simulink model "ieee80211n"  (Simulink 6.0)
settings: Solver=VariableStepDiscrete  StartTime=0.0  StopTime=inf  RelTol=1e-3
PreLoadFcn:
  | load IEEE80211n_init;
values from neighbouring files (symbols this model uses):
  params =     [IEEE80211n_init.mat]    (also in IEEE80211n_settings.m = p)
undefined symbols (not defined in the file or in its folder): magnitude
libraries: commblkintrlv2 x196, dspsigops x143, simulink x136, commdigbbndam2 x98, dspmtrx3 x96, dspsigattribs x69, dspstat3 x38, commutil2 x32, commsequence2 x26, commcnvcod2 x10, dspindex x9, dspmlti3 x8
(part 5 of 12)

== system ieee80211n/ModulatorBank/ModulatorSS1 ==
  mode : Inport  Port=1  LatchInput=off
  txbits : Inport  Port=2  LatchInput=off
  Fcn2 : Fcn  Expr=u==1
  Fcn3 : Fcn  Expr=u==2
  Fcn4 : Fcn  Expr=u==3
  Fcn5 : Fcn  Expr=u==4
  Fcn6 : Fcn  Expr=u==5
  Fcn7 : Fcn  Expr=u==6
  Fcn8 : Fcn  Expr=u==7
  Fcn9 : Fcn  Expr=u==8
  Merge1 : Merge  Inputs=8
  Modulator 1 : Subsystem  AncestorBlock=IEEE80211a_lib/Modulator  TreatAsAtomicUnit=on  mask(QAM Modulator-Coder.){numSymbols=832, modulation=BPSK, code=1/2, trellisStructure=poly2trellis(7, [171 133]), punctureVector=[1]}
      mask prompts: numSymbols "Number of symbols per frame:"; trellisStructure "Trellis:"; punctureVector "Puncture vector:"
      mask help: Modulator gates incoming bits so that a bank of different modulators can share the same input frame size.
      mask init: same as ieee80211n/Demodbank/DecodeBankViterbi/Demodulator 2
      mask Display: disp(['Modulator\n' modulation ' ' code])
  Modulator 2 : Subsystem  AncestorBlock=IEEE80211a_lib/Modulator  TreatAsAtomicUnit=on  mask(QAM Modulator-Coder.){numSymbols=832, modulation=QPSK, code=1/2, trellisStructure=poly2trellis(7, [171 133]), punctureVector=[1]}
      mask prompts: numSymbols "Number of symbols per frame:"; trellisStructure "Trellis:"; punctureVector "Puncture vector:"
      mask help: Modulator gates incoming bits so that a bank of different modulators can share the same input frame size.
      mask init: same as ieee80211n/Demodbank/DecodeBankViterbi/Demodulator 2
      mask Display: disp(['Modulator\n' modulation ' ' code])
  Modulator 3 : Subsystem  AncestorBlock=IEEE80211a_lib/Modulator  TreatAsAtomicUnit=on  mask(QAM Modulator-Coder.){numSymbols=832, modulation=QPSK, code=3/4, trellisStructure=poly2trellis(7, [171 133]), punctureVector=[1 1 1 0 0 1].'}
      mask prompts: numSymbols "Number of symbols per frame:"; trellisStructure "Trellis:"; punctureVector "Puncture vector:"
      mask help: Modulator gates incoming bits so that a bank of different modulators can share the same input frame size.
      mask init: same as ieee80211n/Demodbank/DecodeBankViterbi/Demodulator 2
      mask Display: disp(['Modulator\n' modulation ' ' code])
  Modulator 4 : Subsystem  AncestorBlock=IEEE80211a_lib/Modulator  TreatAsAtomicUnit=on  mask(QAM Modulator-Coder.){numSymbols=832, modulation=16-QAM, code=1/2, trellisStructure=poly2trellis(7, [171 133]), punctureVector=[1]}
      mask prompts: numSymbols "Number of symbols per frame:"; trellisStructure "Trellis:"; punctureVector "Puncture vector:"
      mask help: Modulator gates incoming bits so that a bank of different modulators can share the same input frame size.
      mask init: same as ieee80211n/Demodbank/DecodeBankViterbi/Demodulator 2
      mask Display: disp(['Modulator\n' modulation ' ' code])
  Modulator 5 : Subsystem  AncestorBlock=IEEE80211a_lib/Modulator  TreatAsAtomicUnit=on  mask(QAM Modulator-Coder.){numSymbols=832, modulation=16-QAM, code=3/4, trellisStructure=poly2trellis(7, [171 133]), punctureVector=[1 1 1 0 0 1].'}
      mask prompts: numSymbols "Number of symbols per frame:"; trellisStructure "Trellis:"; punctureVector "Puncture vector:"
      mask help: Modulator gates incoming bits so that a bank of different modulators can share the same input frame size.
      mask init:
      | % number of bits per symbol
      | switch modulation
      | 	case 'BPSK', Nb1 = 1;
      | 	case 'QPSK', Nb1 = 2;
      | 	case '16-QAM', Nb1 = 4;
      | 	case '64-QAM', Nb1 = 6;
      | end
      | 
      | modOrder = 2.^Nb1;
      | Nb = numSymbols * Nb1; % tx bits per block
      | codeRate = str2num(strvcat(code)).';
      | bitsPerBlock = Nb .* codeRate;
      | 
      | % interleaver
      | interleaverRows = 13;
      | if rem(Nb, interleaverRows)
      | 	error('Number of transmitted bits per block must be multiple of 16.')
      | end
      | interleaverCols = Nb / interleaverRows;
      | interleaverElements = [...
      |             2*floor( [0:Nb-1]/2 ) + ...
      |             mod( ([0:Nb-1] + Nb - floor( interleaverRows*[0:Nb-1]/Nb ) ), 2 ) ...
      |             + 1]';
      mask Display: disp(['Modulator\n' modulation ' ' code])
  Modulator 6 : Subsystem  AncestorBlock=IEEE80211a_lib/Modulator  TreatAsAtomicUnit=on  mask(QAM Modulator-Coder.){numSymbols=832, modulation=64-QAM, code=2/3, trellisStructure=poly2trellis(7, [133 171]), punctureVector=[1 1 1 0].'}
      mask prompts: numSymbols "Number of symbols per frame:"; trellisStructure "Trellis:"; punctureVector "Puncture vector:"
      mask help: Modulator gates incoming bits so that a bank of different modulators can share the same input frame size.
      mask init: same as ieee80211n/Demodbank/DecodeBankViterbi/Demodulator 2
      mask Display: disp(['Modulator\n' modulation ' ' code])
  Modulator 7 : Subsystem  AncestorBlock=IEEE80211a_lib/Modulator  TreatAsAtomicUnit=on  mask(QAM Modulator-Coder.){numSymbols=832, modulation=64-QAM, code=3/4, trellisStructure=poly2trellis(7, [133 171]), punctureVector=[1 1 1 0 0 1].'}
      mask prompts: numSymbols "Number of symbols per frame:"; trellisStructure "Trellis:"; punctureVector "Puncture vector:"
      mask help: Modulator gates incoming bits so that a bank of different modulators can share the same input frame size.
      mask init: same as ieee80211n/Demodbank/DecodeBankViterbi/Demodulator 1
      mask Display: disp(['Modulator\n' modulation ' ' code])
  Modulator 8 : Subsystem  AncestorBlock=IEEE80211a_lib/Modulator  TreatAsAtomicUnit=on  mask(QAM Modulator-Coder.){numSymbols=832, modulation=64-QAM, code=5/6, trellisStructure=poly2trellis(7, [133 171]), punctureVector=[1 1 1 0 0 1 1 0 0 1].'}
      mask prompts: numSymbols "Number of symbols per frame:"; trellisStructure "Trellis:"; punctureVector "Puncture vector:"
      mask help: Modulator gates incoming bits so that a bank of different modulators can share the same input frame size.
      mask init: same as ieee80211n/Demodbank/DecodeBankViterbi/Demodulator 2
      mask Display: disp(['Modulator\n' modulation ' ' code])
  sig : Outport
  wires:
  Merge1/1 -> sig/1
  mode/1 -> Fcn2/1, Fcn7/1, Fcn8/1, Fcn9/1, Fcn6/1, Fcn5/1, Fcn4/1, Fcn3/1
  txbits/1 -> Modulator 1/1(txdata), Modulator 6/1(txdata), Modulator 7/1(txdata), Modulator 8/1(txdata), Modulator 5/1(txdata), Modulator 4/1(txdata), Modulator 3/1(txdata), Modulator 2/1(txdata)
  Modulator 1/1(txsig) -> Merge1/1
  Modulator 2/1(txsig) -> Merge1/2
  Modulator 3/1(txsig) -> Merge1/3
  Modulator 4/1(txsig) -> Merge1/4
  Modulator 5/1(txsig) -> Merge1/5
  Modulator 6/1(txsig) -> Merge1/6
  Modulator 7/1(txsig) -> Merge1/7
  Fcn2/1 -> Modulator 1/Enable
  Fcn3/1 -> Modulator 2/Enable
  Fcn4/1 -> Modulator 3/Enable
  Fcn5/1 -> Modulator 4/Enable
  Fcn6/1 -> Modulator 5/Enable
  Fcn7/1 -> Modulator 6/Enable
  Fcn8/1 -> Modulator 7/Enable
  Fcn9/1 -> Modulator 8/Enable
  Modulator 8/1(txsig) -> Merge1/8

== system ieee80211n/ModulatorBank/ModulatorSS2 ==
  mode : Inport  Port=1  LatchInput=off
  txbits : Inport  Port=2  LatchInput=off
  Fcn2 : Fcn  Expr=u==1
  Fcn3 : Fcn  Expr=u==2
  Fcn4 : Fcn  Expr=u==3
  Fcn5 : Fcn  Expr=u==4
  Fcn6 : Fcn  Expr=u==5
  Fcn7 : Fcn  Expr=u==6
  Fcn8 : Fcn  Expr=u==7
  Fcn9 : Fcn  Expr=u==8
  Merge1 : Merge  Inputs=8
  Modulator 1 : Subsystem  AncestorBlock=IEEE80211a_lib/Modulator  TreatAsAtomicUnit=on  mask(QAM Modulator-Coder.){numSymbols=832, modulation=BPSK, code=1/2, trellisStructure=poly2trellis(7, [171 133]), punctureVector=[1]}
      mask prompts: numSymbols "Number of symbols per frame:"; trellisStructure "Trellis:"; punctureVector "Puncture vector:"
      mask help: Modulator gates incoming bits so that a bank of different modulators can share the same input frame size.
      mask init:
      | % number of bits per symbol
      | switch modulation
      | 	case 'BPSK', Nb1 = 1;
      | 	case 'QPSK', Nb1 = 2;
      | 	case '16-QAM', Nb1 = 4;
      | 	case '64-QAM', Nb1 = 6;
      | end
      | 
      | modOrder = 2.^Nb1;
      | Nb = numSymbols * Nb1; % tx bits per block
      | codeRate = str2num(strvcat(code)).';
      | bitsPerBlock = Nb .* codeRate;
      | s=max([Nb1/2 1]);
      | 
      | % interleaver
      | interleaverRows = 13;
      | if rem(Nb, interleaverRows)
      | 	error('Number of transmitted bits per block must be multiple of 16.')
      | end
      | interleaverCols = Nb / interleaverRows;
      | interleaverElements = [...
      |             s*floor( [0:Nb-1]/s ) + ...
      |             mod( ([0:Nb-1] + Nb - floor( interleaverRows*[0:Nb-1]/Nb ) ), s ) ...
      |             + 1]';
      | 	
      | if 1 %%%%%%%%%%%%%%%%%%%%%%%%
      | % freq rotation interleaver
      | iss = 1;
      | freqRotNum = 2*11;  % 20MHz channel
      | freqRotInterleaverElements = [...
      |             mod([0:Nb-1] - (mod(2*iss, 3) + 3*floor(iss/3)*freqRotNum*Nb1), Nb) ...
      |             + 1]';
      | end   %%%%%%%%%%%%%%%%%%%%%%%%
      mask Display: disp(['Modulator\n' modulation ' ' code])
  Modulator 2 : Subsystem  AncestorBlock=IEEE80211a_lib/Modulator  TreatAsAtomicUnit=on  mask(QAM Modulator-Coder.){numSymbols=832, modulation=QPSK, code=1/2, trellisStructure=poly2trellis(7, [171 133]), punctureVector=[1]}
      mask prompts: numSymbols "Number of symbols per frame:"; trellisStructure "Trellis:"; punctureVector "Puncture vector:"
      mask help: Modulator gates incoming bits so that a bank of different modulators can share the same input frame size.
      mask init: same as ieee80211n/Demodbank/Demod_ss2/Demodulator 1
      mask Display: disp(['Modulator\n' modulation ' ' code])
  Modulator 3 : Subsystem  AncestorBlock=IEEE80211a_lib/Modulator  TreatAsAtomicUnit=on  mask(QAM Modulator-Coder.){numSymbols=832, modulation=QPSK, code=3/4, trellisStructure=poly2trellis(7, [171 133]), punctureVector=[1 1 1 0 0 1].'}
      mask prompts: numSymbols "Number of symbols per frame:"; trellisStructure "Trellis:"; punctureVector "Puncture vector:"
      mask help: Modulator gates incoming bits so that a bank of different modulators can share the same input frame size.
      mask init: same as ieee80211n/Demodbank/Demod_ss2/Demodulator 1
      mask Display: disp(['Modulator\n' modulation ' ' code])
  Modulator 4 : Subsystem  AncestorBlock=IEEE80211a_lib/Modulator  TreatAsAtomicUnit=on  mask(QAM Modulator-Coder.){numSymbols=832, modulation=16-QAM, code=1/2, trellisStructure=poly2trellis(7, [171 133]), punctureVector=[1]}
      mask prompts: numSymbols "Number of symbols per frame:"; trellisStructure "Trellis:"; punctureVector "Puncture vector:"
      mask help: Modulator gates incoming bits so that a bank of different modulators can share the same input frame size.
      mask init: same as ieee80211n/Demodbank/Demod_ss2/Demodulator 1
      mask Display: disp(['Modulator\n' modulation ' ' code])
  Modulator 5 : Subsystem  AncestorBlock=IEEE80211a_lib/Modulator  TreatAsAtomicUnit=on  mask(QAM Modulator-Coder.){numSymbols=832, modulation=16-QAM, code=3/4, trellisStructure=poly2trellis(7, [171 133]), punctureVector=[1 1 1 0 0 1].'}
      mask prompts: numSymbols "Number of symbols per frame:"; trellisStructure "Trellis:"; punctureVector "Puncture vector:"
      mask help: Modulator gates incoming bits so that a bank of different modulators can share the same input frame size.
      mask init: same as ieee80211n/Demodbank/Demod_ss2/Demodulator 1
      mask Display: disp(['Modulator\n' modulation ' ' code])
  Modulator 6 : Subsystem  AncestorBlock=IEEE80211a_lib/Modulator  TreatAsAtomicUnit=on  mask(QAM Modulator-Coder.){numSymbols=832, modulation=64-QAM, code=2/3, trellisStructure=poly2trellis(7, [133 171]), punctureVector=[1 1 1 0].'}
      mask prompts: numSymbols "Number of symbols per frame:"; trellisStructure "Trellis:"; punctureVector "Puncture vector:"
      mask help: Modulator gates incoming bits so that a bank of different modulators can share the same input frame size.
      mask init: same as ieee80211n/Demodbank/Demod_ss2/Demodulator 1
      mask Display: disp(['Modulator\n' modulation ' ' code])
  Modulator 7 : Subsystem  AncestorBlock=IEEE80211a_lib/Modulator  TreatAsAtomicUnit=on  mask(QAM Modulator-Coder.){numSymbols=832, modulation=64-QAM, code=3/4, trellisStructure=poly2trellis(7, [133 171]), punctureVector=[1 1 1 0 0 1].'}
      mask prompts: numSymbols "Number of symbols per frame:"; trellisStructure "Trellis:"; punctureVector "Puncture vector:"
      mask help: Modulator gates incoming bits so that a bank of different modulators can share the same input frame size.
      mask init: same as ieee80211n/Demodbank/Demod_ss2/Demodulator 1
      mask Display: disp(['Modulator\n' modulation ' ' code])
  Modulator 8 : Subsystem  AncestorBlock=IEEE80211a_lib/Modulator  TreatAsAtomicUnit=on  mask(QAM Modulator-Coder.){numSymbols=832, modulation=64-QAM, code=5/6, trellisStructure=poly2trellis(7, [133 171]), punctureVector=[1 1 1 0 0 1 1 0 0 1].'}
      mask prompts: numSymbols "Number of symbols per frame:"; trellisStructure "Trellis:"; punctureVector "Puncture vector:"
      mask help: Modulator gates incoming bits so that a bank of different modulators can share the same input frame size.
      mask init:
      | % number of bits per symbol
      | switch modulation
      | 	case 'BPSK', Nb1 = 1;
      | 	case 'QPSK', Nb1 = 2;
      | 	case '16-QAM', Nb1 = 4;
      | 	case '64-QAM', Nb1 = 6;
      | 	case '256-QAM', Nb1 = 8;
      | end
      | 
      | modOrder = 2.^Nb1;
      | Nb = numSymbols * Nb1; % tx bits per block
      | codeRate = str2num(strvcat(code)).';
      | bitsPerBlock = Nb .* codeRate;
      | s=max([Nb1/2 1]);
      | 
      | % interleaver
      | interleaverRows = 13;
      | if rem(Nb, interleaverRows)
      | 	error('Number of transmitted bits per block must be multiple of 16.')
      | end
      | interleaverCols = Nb / interleaverRows;
      | interleaverElements = [...
      |             s*floor( [0:Nb-1]/s ) + ...
      |             mod( ([0:Nb-1] + Nb - floor( interleaverRows*[0:Nb-1]/Nb ) ), s ) ...
      |             + 1]';
      | 	
      | if 1 %%%%%%%%%%%%%%%%%%%%%%%%
      | % freq rotation interleaver
      | iss = 1;
      | freqRotNum = 2*11;  % 20MHz channel
      | freqRotInterleaverElements = [...
      |             mod([0:Nb-1] - (mod(2*iss, 3) + 3*floor(iss/3)*freqRotNum*Nb1), Nb) ...
      |             + 1]';
      | end   %%%%%%%%%%%%%%%%%%%%%%%%
      mask Display: disp(['Modulator\n' modulation ' ' code])
  sig : Outport
  wires:
  Merge1/1 -> sig/1
  mode/1 -> Fcn2/1, Fcn7/1, Fcn8/1, Fcn9/1, Fcn6/1, Fcn5/1, Fcn4/1, Fcn3/1
  txbits/1 -> Modulator 1/1(txdata), Modulator 6/1(txdata), Modulator 7/1(txdata), Modulator 8/1(txdata), Modulator 5/1(txdata), Modulator 4/1(txdata), Modulator 3/1(txdata), Modulator 2/1(txdata)
  Modulator 1/1(txsig) -> Merge1/1
  Modulator 2/1(txsig) -> Merge1/2
  Modulator 3/1(txsig) -> Merge1/3
  Modulator 4/1(txsig) -> Merge1/4
  Modulator 5/1(txsig) -> Merge1/5
  Modulator 6/1(txsig) -> Merge1/6
  Modulator 7/1(txsig) -> Merge1/7
  Fcn2/1 -> Modulator 1/Enable
  Fcn3/1 -> Modulator 2/Enable
  Fcn4/1 -> Modulator 3/Enable
  Fcn5/1 -> Modulator 4/Enable
  Fcn6/1 -> Modulator 5/Enable
  Fcn7/1 -> Modulator 6/Enable
  Fcn8/1 -> Modulator 7/Enable
  Fcn9/1 -> Modulator 8/Enable
  Modulator 8/1(txsig) -> Merge1/8

== system ieee80211n/ModulatorBank/ModulatorSS3 ==
  mode : Inport  Port=1  LatchInput=off
  txbits : Inport  Port=2  LatchInput=off
  Fcn2 : Fcn  Expr=u==1
  Fcn3 : Fcn  Expr=u==2
  Fcn4 : Fcn  Expr=u==3
  Fcn5 : Fcn  Expr=u==4
  Fcn6 : Fcn  Expr=u==5
  Fcn7 : Fcn  Expr=u==6
  Fcn8 : Fcn  Expr=u==7
  Fcn9 : Fcn  Expr=u==8
  Merge1 : Merge  Inputs=8
  Modulator 1 : Subsystem  AncestorBlock=IEEE80211a_lib/Modulator  TreatAsAtomicUnit=on  mask(QAM Modulator-Coder.){numSymbols=832, modulation=BPSK, code=1/2, trellisStructure=poly2trellis(7, [171 133]), punctureVector=[1]}
      mask prompts: numSymbols "Number of symbols per frame:"; trellisStructure "Trellis:"; punctureVector "Puncture vector:"
      mask help: Modulator gates incoming bits so that a bank of different modulators can share the same input frame size.
      mask init:
      | % number of bits per symbol
      | switch modulation
      | 	case 'BPSK', Nb1 = 1;
      | 	case 'QPSK', Nb1 = 2;
      | 	case '16-QAM', Nb1 = 4;
      | 	case '64-QAM', Nb1 = 6;
      | end
      | 
      | modOrder = 2.^Nb1;
      | Nb = numSymbols * Nb1; % tx bits per block
      | codeRate = str2num(strvcat(code)).';
      | bitsPerBlock = Nb .* codeRate;
      | s=max([Nb1/2 1]);
      | 
      | % interleaver
      | interleaverRows = 13;
      | if rem(Nb, interleaverRows)
      | 	error('Number of transmitted bits per block must be multiple of 16.')
      | end
      | interleaverCols = Nb / interleaverRows;
      | interleaverElements = [...
      |             s*floor( [0:Nb-1]/s ) + ...
      |             mod( ([0:Nb-1] + Nb - floor( interleaverRows*[0:Nb-1]/Nb ) ), s ) ...
      |             + 1]';
      | 	
      | if 1 %%%%%%%%%%%%%%%%%%%%%%%%
      | % freq rotation interleaver
      | iss = 2;
      | freqRotNum = 1*11;  % 20MHz channel
      | freqRotInterleaverElements = [...
      |             mod([0:Nb-1] - (mod(2*iss, 3) + 3*floor(iss/3)*freqRotNum*Nb1), Nb) ...
      |             + 1]';
      | end   %%%%%%%%%%%%%%%%%%%%%%%%
      mask Display: disp(['Modulator\n' modulation ' ' code])
  Modulator 2 : Subsystem  AncestorBlock=IEEE80211a_lib/Modulator  TreatAsAtomicUnit=on  mask(QAM Modulator-Coder.){numSymbols=832, modulation=QPSK, code=1/2, trellisStructure=poly2trellis(7, [171 133]), punctureVector=[1]}
      mask prompts: numSymbols "Number of symbols per frame:"; trellisStructure "Trellis:"; punctureVector "Puncture vector:"
      mask help: Modulator gates incoming bits so that a bank of different modulators can share the same input frame size.
      mask init: same as ieee80211n/ModulatorBank/ModulatorSS3/Modulator 1
      mask Display: disp(['Modulator\n' modulation ' ' code])
  Modulator 3 : Subsystem  AncestorBlock=IEEE80211a_lib/Modulator  TreatAsAtomicUnit=on  mask(QAM Modulator-Coder.){numSymbols=832, modulation=QPSK, code=3/4, trellisStructure=poly2trellis(7, [171 133]), punctureVector=[1 1 1 0 0 1].'}
      mask prompts: numSymbols "Number of symbols per frame:"; trellisStructure "Trellis:"; punctureVector "Puncture vector:"
      mask help: Modulator gates incoming bits so that a bank of different modulators can share the same input frame size.
      mask init: same as ieee80211n/ModulatorBank/ModulatorSS3/Modulator 1
      mask Display: disp(['Modulator\n' modulation ' ' code])
  Modulator 4 : Subsystem  AncestorBlock=IEEE80211a_lib/Modulator  TreatAsAtomicUnit=on  mask(QAM Modulator-Coder.){numSymbols=832, modulation=16-QAM, code=1/2, trellisStructure=poly2trellis(7, [171 133]), punctureVector=[1]}
      mask prompts: numSymbols "Number of symbols per frame:"; trellisStructure "Trellis:"; punctureVector "Puncture vector:"
      mask help: Modulator gates incoming bits so that a bank of different modulators can share the same input frame size.
      mask init: same as ieee80211n/ModulatorBank/ModulatorSS3/Modulator 1
      mask Display: disp(['Modulator\n' modulation ' ' code])
  Modulator 5 : Subsystem  AncestorBlock=IEEE80211a_lib/Modulator  TreatAsAtomicUnit=on  mask(QAM Modulator-Coder.){numSymbols=832, modulation=16-QAM, code=3/4, trellisStructure=poly2trellis(7, [171 133]), punctureVector=[1 1 1 0 0 1].'}
      mask prompts: numSymbols "Number of symbols per frame:"; trellisStructure "Trellis:"; punctureVector "Puncture vector:"
      mask help: Modulator gates incoming bits so that a bank of different modulators can share the same input frame size.
      mask init: same as ieee80211n/ModulatorBank/ModulatorSS3/Modulator 1
      mask Display: disp(['Modulator\n' modulation ' ' code])
  Modulator 6 : Subsystem  AncestorBlock=IEEE80211a_lib/Modulator  TreatAsAtomicUnit=on  mask(QAM Modulator-Coder.){numSymbols=832, modulation=64-QAM, code=2/3, trellisStructure=poly2trellis(7, [133 171]), punctureVector=[1 1 1 0].'}
      mask prompts: numSymbols "Number of symbols per frame:"; trellisStructure "Trellis:"; punctureVector "Puncture vector:"
      mask help: Modulator gates incoming bits so that a bank of different modulators can share the same input frame size.
      mask init: same as ieee80211n/ModulatorBank/ModulatorSS3/Modulator 1
      mask Display: disp(['Modulator\n' modulation ' ' code])
  Modulator 7 : Subsystem  AncestorBlock=IEEE80211a_lib/Modulator  TreatAsAtomicUnit=on  mask(QAM Modulator-Coder.){numSymbols=832, modulation=64-QAM, code=3/4, trellisStructure=poly2trellis(7, [133 171]), punctureVector=[1 1 1 0 0 1].'}
      mask prompts: numSymbols "Number of symbols per frame:"; trellisStructure "Trellis:"; punctureVector "Puncture vector:"
      mask help: Modulator gates incoming bits so that a bank of different modulators can share the same input frame size.
      mask init: same as ieee80211n/ModulatorBank/ModulatorSS3/Modulator 1
      mask Display: disp(['Modulator\n' modulation ' ' code])
  Modulator 8 : Subsystem  AncestorBlock=IEEE80211a_lib/Modulator  TreatAsAtomicUnit=on  mask(QAM Modulator-Coder.){numSymbols=832, modulation=64-QAM, code=5/6, trellisStructure=poly2trellis(7, [133 171]), punctureVector=[1 1 1 0 0 1 1 0 0 1].'}
      mask prompts: numSymbols "Number of symbols per frame:"; trellisStructure "Trellis:"; punctureVector "Puncture vector:"
      mask help: Modulator gates incoming bits so that a bank of different modulators can share the same input frame size.
      mask init:
      | % number of bits per symbol
      | switch modulation
      | 	case 'BPSK', Nb1 = 1;
      | 	case 'QPSK', Nb1 = 2;
      | 	case '16-QAM', Nb1 = 4;
      | 	case '64-QAM', Nb1 = 6;
      | 	case '256-QAM', Nb1 = 8;
      | end
      | 
      | modOrder = 2.^Nb1;
      | Nb = numSymbols * Nb1; % tx bits per block
      | codeRate = str2num(strvcat(code)).';
      | bitsPerBlock = Nb .* codeRate;
      | s=max([Nb1/2 1]);
      | 
      | % interleaver
      | interleaverRows = 13;
      | if rem(Nb, interleaverRows)
      | 	error('Number of transmitted bits per block must be multiple of 16.')
      | end
      | interleaverCols = Nb / interleaverRows;
      | interleaverElements = [...
      |             s*floor( [0:Nb-1]/s ) + ...
      |             mod( ([0:Nb-1] + Nb - floor( interleaverRows*[0:Nb-1]/Nb ) ), s ) ...
      |             + 1]';
      | 	
      | if 1 %%%%%%%%%%%%%%%%%%%%%%%%
      | % freq rotation interleaver
      | iss = 2;
      | freqRotNum = 1*11;  % 20MHz channel
      | freqRotInterleaverElements = [...
      |             mod([0:Nb-1] - (mod(2*iss, 3) + 3*floor(iss/3)*freqRotNum*Nb1), Nb) ...
      |             + 1]';
      | end   %%%%%%%%%%%%%%%%%%%%%%%%
      mask Display: disp(['Modulator\n' modulation ' ' code])
  sig : Outport
  wires:
  Merge1/1 -> sig/1
  mode/1 -> Fcn2/1, Fcn7/1, Fcn8/1, Fcn9/1, Fcn6/1, Fcn5/1, Fcn4/1, Fcn3/1
  txbits/1 -> Modulator 1/1(txdata), Modulator 6/1(txdata), Modulator 7/1(txdata), Modulator 8/1(txdata), Modulator 5/1(txdata), Modulator 4/1(txdata), Modulator 3/1(txdata), Modulator 2/1(txdata)
  Modulator 1/1(txsig) -> Merge1/1
  Modulator 2/1(txsig) -> Merge1/2
  Modulator 3/1(txsig) -> Merge1/3
  Modulator 4/1(txsig) -> Merge1/4
  Modulator 5/1(txsig) -> Merge1/5
  Modulator 6/1(txsig) -> Merge1/6
  Modulator 7/1(txsig) -> Merge1/7
  Fcn2/1 -> Modulator 1/Enable
  Fcn3/1 -> Modulator 2/Enable
  Fcn4/1 -> Modulator 3/Enable
  Fcn5/1 -> Modulator 4/Enable
  Fcn6/1 -> Modulator 5/Enable
  Fcn7/1 -> Modulator 6/Enable
  Fcn8/1 -> Modulator 7/Enable
  Fcn9/1 -> Modulator 8/Enable
  Modulator 8/1(txsig) -> Merge1/8

== system ieee80211n/ModulatorBank/ModulatorSS4 ==
  mode : Inport  Port=1  LatchInput=off
  txbits : Inport  Port=2  LatchInput=off
  Fcn2 : Fcn  Expr=u==1
  Fcn3 : Fcn  Expr=u==2
  Fcn4 : Fcn  Expr=u==3
  Fcn5 : Fcn  Expr=u==4
  Fcn6 : Fcn  Expr=u==5
  Fcn7 : Fcn  Expr=u==6
  Fcn8 : Fcn  Expr=u==7
  Fcn9 : Fcn  Expr=u==8
  Merge1 : Merge  Inputs=8
  Modulator 1 : Subsystem  AncestorBlock=IEEE80211a_lib/Modulator  TreatAsAtomicUnit=on  mask(QAM Modulator-Coder.){numSymbols=832, modulation=BPSK, code=1/2, trellisStructure=poly2trellis(7, [171 133]), punctureVector=[1]}
      mask prompts: numSymbols "Number of symbols per frame:"; trellisStructure "Trellis:"; punctureVector "Puncture vector:"
      mask help: Modulator gates incoming bits so that a bank of different modulators can share the same input frame size.
      mask init:
      | % number of bits per symbol
      | switch modulation
      | 	case 'BPSK', Nb1 = 1;
      | 	case 'QPSK', Nb1 = 2;
      | 	case '16-QAM', Nb1 = 4;
      | 	case '64-QAM', Nb1 = 6;
      | end
      | 
      | modOrder = 2.^Nb1;
      | Nb = numSymbols * Nb1; % tx bits per block
      | codeRate = str2num(strvcat(code)).';
      | bitsPerBlock = Nb .* codeRate;
      | s=max([Nb1/2 1]);
      | 
      | % interleaver
      | interleaverRows = 13;
      | if rem(Nb, interleaverRows)
      | 	error('Number of transmitted bits per block must be multiple of 16.')
      | end
      | interleaverCols = Nb / interleaverRows;
      | interleaverElements = [...
      |             s*floor( [0:Nb-1]/s ) + ...
      |             mod( ([0:Nb-1] + Nb - floor( interleaverRows*[0:Nb-1]/Nb ) ), s ) ...
      |             + 1]';
      | 	
      | if 1 %%%%%%%%%%%%%%%%%%%%%%%%
      | % freq rotation interleaver
      | iss = 3;
      | freqRotNum = 3*11;  % 20MHz channel
      | freqRotInterleaverElements = [...
      |             mod([0:Nb-1] - (mod(2*iss, 3) + 3*floor(iss/3)*freqRotNum*Nb1), Nb) ...
      |             + 1]';
      | end   %%%%%%%%%%%%%%%%%%%%%%%%
      mask Display: disp(['Modulator\n' modulation ' ' code])
  Modulator 2 : Subsystem  AncestorBlock=IEEE80211a_lib/Modulator  TreatAsAtomicUnit=on  mask(QAM Modulator-Coder.){numSymbols=832, modulation=QPSK, code=1/2, trellisStructure=poly2trellis(7, [171 133]), punctureVector=[1]}
      mask prompts: numSymbols "Number of symbols per frame:"; trellisStructure "Trellis:"; punctureVector "Puncture vector:"
      mask help: Modulator gates incoming bits so that a bank of different modulators can share the same input frame size.
      mask init: same as ieee80211n/Demodbank/Demod_ss4/Demodulator 1
      mask Display: disp(['Modulator\n' modulation ' ' code])
  Modulator 3 : Subsystem  AncestorBlock=IEEE80211a_lib/Modulator  TreatAsAtomicUnit=on  mask(QAM Modulator-Coder.){numSymbols=832, modulation=QPSK, code=3/4, trellisStructure=poly2trellis(7, [171 133]), punctureVector=[1 1 1 0 0 1].'}
      mask prompts: numSymbols "Number of symbols per frame:"; trellisStructure "Trellis:"; punctureVector "Puncture vector:"
      mask help: Modulator gates incoming bits so that a bank of different modulators can share the same input frame size.
      mask init: same as ieee80211n/Demodbank/Demod_ss4/Demodulator 1
      mask Display: disp(['Modulator\n' modulation ' ' code])
  Modulator 4 : Subsystem  AncestorBlock=IEEE80211a_lib/Modulator  TreatAsAtomicUnit=on  mask(QAM Modulator-Coder.){numSymbols=832, modulation=16-QAM, code=1/2, trellisStructure=poly2trellis(7, [171 133]), punctureVector=[1]}
      mask prompts: numSymbols "Number of symbols per frame:"; trellisStructure "Trellis:"; punctureVector "Puncture vector:"
      mask help: Modulator gates incoming bits so that a bank of different modulators can share the same input frame size.
      mask init: same as ieee80211n/Demodbank/Demod_ss4/Demodulator 1
      mask Display: disp(['Modulator\n' modulation ' ' code])
  Modulator 5 : Subsystem  AncestorBlock=IEEE80211a_lib/Modulator  TreatAsAtomicUnit=on  mask(QAM Modulator-Coder.){numSymbols=832, modulation=16-QAM, code=3/4, trellisStructure=poly2trellis(7, [171 133]), punctureVector=[1 1 1 0 0 1].'}
      mask prompts: numSymbols "Number of symbols per frame:"; trellisStructure "Trellis:"; punctureVector "Puncture vector:"
      mask help: Modulator gates incoming bits so that a bank of different modulators can share the same input frame size.
      mask init: same as ieee80211n/Demodbank/Demod_ss4/Demodulator 1
      mask Display: disp(['Modulator\n' modulation ' ' code])
  Modulator 6 : Subsystem  AncestorBlock=IEEE80211a_lib/Modulator  TreatAsAtomicUnit=on  mask(QAM Modulator-Coder.){numSymbols=832, modulation=64-QAM, code=2/3, trellisStructure=poly2trellis(7, [133 171]), punctureVector=[1 1 1 0].'}
      mask prompts: numSymbols "Number of symbols per frame:"; trellisStructure "Trellis:"; punctureVector "Puncture vector:"
      mask help: Modulator gates incoming bits so that a bank of different modulators can share the same input frame size.
      mask init: same as ieee80211n/Demodbank/Demod_ss4/Demodulator 1
      mask Display: disp(['Modulator\n' modulation ' ' code])
  Modulator 7 : Subsystem  AncestorBlock=IEEE80211a_lib/Modulator  TreatAsAtomicUnit=on  mask(QAM Modulator-Coder.){numSymbols=832, modulation=64-QAM, code=3/4, trellisStructure=poly2trellis(7, [133 171]), punctureVector=[1 1 1 0 0 1].'}
      mask prompts: numSymbols "Number of symbols per frame:"; trellisStructure "Trellis:"; punctureVector "Puncture vector:"
      mask help: Modulator gates incoming bits so that a bank of different modulators can share the same input frame size.
      mask init: same as ieee80211n/Demodbank/Demod_ss4/Demodulator 1
      mask Display: disp(['Modulator\n' modulation ' ' code])
  Modulator 8 : Subsystem  AncestorBlock=IEEE80211a_lib/Modulator  TreatAsAtomicUnit=on  mask(QAM Modulator-Coder.){numSymbols=832, modulation=64-QAM, code=5/6, trellisStructure=poly2trellis(7, [133 171]), punctureVector=[1 1 1 0 0 1 1 0 0 1].'}
      mask prompts: numSymbols "Number of symbols per frame:"; trellisStructure "Trellis:"; punctureVector "Puncture vector:"
      mask help: Modulator gates incoming bits so that a bank of different modulators can share the same input frame size.
      mask init:
      | % number of bits per symbol
      | switch modulation
      | 	case 'BPSK', Nb1 = 1;
      | 	case 'QPSK', Nb1 = 2;
      | 	case '16-QAM', Nb1 = 4;
      | 	case '64-QAM', Nb1 = 6;
      | 	case '256-QAM', Nb1 = 8;
      | end
      | 
      | modOrder = 2.^Nb1;
      | Nb = numSymbols * Nb1; % tx bits per block
      | codeRate = str2num(strvcat(code)).';
      | bitsPerBlock = Nb .* codeRate;
      | s=max([Nb1/2 1]);
      | 
      | % interleaver
      | interleaverRows = 13;
      | if rem(Nb, interleaverRows)
      | 	error('Number of transmitted bits per block must be multiple of 16.')
      | end
      | interleaverCols = Nb / interleaverRows;
      | interleaverElements = [...
      |             s*floor( [0:Nb-1]/s ) + ...
      |             mod( ([0:Nb-1] + Nb - floor( interleaverRows*[0:Nb-1]/Nb ) ), s ) ...
      |             + 1]';
      | 	
      | if 1 %%%%%%%%%%%%%%%%%%%%%%%%
      | % freq rotation interleaver
      | iss = 3;
      | freqRotNum = 3*11;  % 20MHz channel
      | freqRotInterleaverElements = [...
      |             mod([0:Nb-1] - (mod(2*iss, 3) + 3*floor(iss/3)*freqRotNum*Nb1), Nb) ...
      |             + 1]';
      | end   %%%%%%%%%%%%%%%%%%%%%%%%
      mask Display: disp(['Modulator\n' modulation ' ' code])
  sig : Outport
  wires:
  Merge1/1 -> sig/1
  mode/1 -> Fcn2/1, Fcn7/1, Fcn8/1, Fcn9/1, Fcn6/1, Fcn5/1, Fcn4/1, Fcn3/1
  txbits/1 -> Modulator 1/1(txdata), Modulator 6/1(txdata), Modulator 7/1(txdata), Modulator 8/1(txdata), Modulator 5/1(txdata), Modulator 4/1(txdata), Modulator 3/1(txdata), Modulator 2/1(txdata)
  Modulator 1/1(txsig) -> Merge1/1
  Modulator 2/1(txsig) -> Merge1/2
  Modulator 3/1(txsig) -> Merge1/3
  Modulator 4/1(txsig) -> Merge1/4
  Modulator 5/1(txsig) -> Merge1/5
  Modulator 6/1(txsig) -> Merge1/6
  Modulator 7/1(txsig) -> Merge1/7
  Fcn2/1 -> Modulator 1/Enable
  Fcn3/1 -> Modulator 2/Enable
  Fcn4/1 -> Modulator 3/Enable
  Fcn5/1 -> Modulator 4/Enable
  Fcn6/1 -> Modulator 5/Enable
  Fcn7/1 -> Modulator 6/Enable
  Fcn8/1 -> Modulator 7/Enable
  Fcn9/1 -> Modulator 8/Enable
  Modulator 8/1(txsig) -> Merge1/8

== system ieee80211n/PER calculation/Bit indices ==
  mode : Inport  Port=1  LatchInput=off
  delay : Inport  Port=2  LatchInput=off
  Constant : Constant  Value=(1:params.NSS*max(params.bitsPerBlock)).'  VectorParams1D=off
  Product : Product  Inputs=3  SaturateOnIntegerOverflow=on
  Relational Operator1 : RelationalOperator  Operator=<=  LogicOutDataTypeMode=Specify via dialog  LogicDataType=float('double')  InputSameDT=on
  Relational Operator2 : RelationalOperator  Operator=>  LogicOutDataTypeMode=Specify via dialog  LogicDataType=float('double')  InputSameDT=on
  bits per block : IEEE80211a_lib/Select value  vector=params.NSS*params.bitsPerBlock.'
  sel : Outport
  wires:
  Relational Operator1/1 -> Product/2
  Relational Operator2/1 -> Product/3
  delay/1 -> Relational Operator2/2
  Product/1 -> sel/1
  bits per block/1 -> Relational Operator1/2
  Constant/1 -> Relational Operator1/1, Relational Operator2/1, Product/1
  mode/1 -> bits per block/1

== system ieee80211n/PER calculation/Translate to packet error rate ==
  note: Packet error rate taken over last 50 frames
  note: bit errors in
      | current pkt
  note: packet errors
  note: num packets
  bit errors : Inport  Port=1  LatchInput=off
  Constant : Constant  Value=0
  Convert to % : Gain  Gain=100  SaturateOnIntegerOverflow=on
  Data Type Conversion : DataTypeConversion  OutDataTypeMode=double  SaturateOnIntegerOverflow=on  RndMeth=Zero
  Fcn : Fcn  Expr=1
  Integer Delay : dspobslib/Integer Delay  delay=1  ic=0  reset_popup=None
  Integer Delay1 : dspobslib/Integer Delay  Orientation=left  delay=1  ic=0  reset_popup=None
  Integer Delay2 : dspobslib/Integer Delay  Orientation=left  delay=1  ic=0  reset_popup=None
  Integer Delay3 : dspobslib/Integer Delay  delay=50  ic=0  reset_popup=None
  Integer Delay4 : dspobslib/Integer Delay  delay=50  ic=0  reset_popup=None
  Product : Product  Inputs=*/  SaturateOnIntegerOverflow=on
  Relational Operator : RelationalOperator  Operator=>
  Rounding Function : Rounding  Operator=round
  Rounding Function1 : Rounding  Operator=round
  Rounding Function2 : Rounding  Operator=round
  Sum : Sum  Inputs=|+-  SaturateOnIntegerOverflow=on
  Sum1 : Sum  Inputs=+-+  SaturateOnIntegerOverflow=on
  Sum2 : Sum  Inputs=+-+  SaturateOnIntegerOverflow=on
  PER : Outport
  wires:
  Rounding Function2/1 -> Integer Delay2/1, Product/2
  Rounding Function1/1 -> Integer Delay1/1, Product/1
  Rounding Function/1 -> PER/1
  Sum1/1 -> Rounding Function1/1
  Integer Delay1/1 -> Sum1/3
  Integer Delay3/1 -> Sum1/2
  Data Type Conversion/1 -> Sum1/1, Integer Delay3/1
  Integer Delay2/1 -> Sum2/3
  Integer Delay4/1 -> Sum2/2
  Sum2/1 -> Rounding Function2/1
  bit errors/1 -> Fcn/1, Integer Delay/1, Sum/1
  Convert to %/1 -> Rounding Function/1
  Product/1 -> Convert to %/1
  Fcn/1 -> Integer Delay4/1, Sum2/1
  Constant/1 -> Relational Operator/2
  Relational Operator/1 -> Data Type Conversion/1
  Sum/1 -> Relational Operator/1
  Integer Delay/1 -> Sum/2

== system ieee80211n/cyclic prefix/Cyclic shift, SS1 ==
  in : Inport  Port=1  LatchInput=off
  HT Cyclic Shift : Selector  InputType=Matrix  Elements=[49:64 1:64]  Rows=params.cs2_HT20_ss1  Columns=-1  InputPortWidth=64
  HT-STF Cyclic Shift : Selector  InputType=Matrix  Elements=[49:64 1:64]  Rows=params.cs2_HT20_STF_ss1  Columns=-1  InputPortWidth=64
  Legacy Cyclic Shift : Selector  InputType=Matrix  Elements=[49:64 1:64]  Rows=params.cs2_Legacy_ss1  Columns=-1  InputPortWidth=64
  Merge Legacy/HT : simulink/Math Operations/Matrix Concatenation  numInports=3  catMethod=Horizontal
  "Train/Data, SS1" : S-Function  AncestorBlock=dspindex/Multiport Selector  FunctionName=sdspmultiportsel  Parameters=rowsOrCols, numOutports, flatIdxVect, flatLenVect, idxErrMode  mask(Multiport Selector){rowsOrCols=Columns, idxCellArray={params.cs2_Indices1, params.cs2_Indices2, params.cs2_Indices3}, idxErrMode=Clip Index}
      mask prompts: rowsOrCols "Select:"; idxCellArray "Indices to output:"; idxErrMode "Invalid index:"
      mask help: Output specified rows or columns to one or more output ports. The number of output ports is determined by the number of index vectors, each specified as a separate vector entry in a cell array. Indices are 1-based and need not be unique.
      mask init:
      | [numOutports, flatLenVect, flatIdxVect] = dspblkmultiportsel(idxCellArray);
      mask Help: web(dspbhelp);
      mask StyleString: popup(Rows|Columns),edit,popup(Clip Index|Clip and Warn|Generate Error)
      mask Display: disp(['Select\n' &1]);
  out : Outport
  wires:
  "Train/Data, SS1"/1 -> Legacy Cyclic Shift/1
  "Train/Data, SS1"/2 -> HT-STF Cyclic Shift/1
  Legacy Cyclic Shift/1 -> Merge Legacy/HT/1
  HT-STF Cyclic Shift/1 -> Merge Legacy/HT/2
  Merge Legacy/HT/1 -> out/1
  in/1 -> "Train/Data, SS1"/1
  "Train/Data, SS1"/3 -> HT Cyclic Shift/1
  HT Cyclic Shift/1 -> Merge Legacy/HT/3

== system ieee80211n/cyclic prefix1/Cyclic shift, SS2 ==
  in : Inport  Port=1  LatchInput=off
  HT Cyclic Shift : Selector  InputType=Matrix  Elements=[49:64 1:64]  Rows=params.cs2_HT20_ss2  Columns=-1  InputPortWidth=64
  HT-STF Cyclic Shift : Selector  InputType=Matrix  Elements=[49:64 1:64]  Rows=params.cs2_HT20_STF_ss2  Columns=-1  InputPortWidth=64
  Legacy Cyclic Shift : Selector  InputType=Matrix  Elements=[49:64 1:64]  Rows=params.cs2_Legacy_ss2  Columns=-1  InputPortWidth=64
  Merge Legacy/HT : simulink/Math Operations/Matrix Concatenation  numInports=3  catMethod=Horizontal
  "Train/Data, SS2" : S-Function  AncestorBlock=dspindex/Multiport Selector  FunctionName=sdspmultiportsel  Parameters=rowsOrCols, numOutports, flatIdxVect, flatLenVect, idxErrMode  mask(Multiport Selector){rowsOrCols=Columns, idxCellArray={params.cs2_Indices1,params.cs2_Indices2,params.cs2_Indices3}, idxErrMode=Clip Index}
      mask prompts: rowsOrCols "Select:"; idxCellArray "Indices to output:"; idxErrMode "Invalid index:"
      mask help: Output specified rows or columns to one or more output ports. The number of output ports is determined by the number of index vectors, each specified as a separate vector entry in a cell array. Indices are 1-based and need not be unique.
      mask init:
      | [numOutports, flatLenVect, flatIdxVect] = dspblkmultiportsel(idxCellArray);
      mask Help: web(dspbhelp);
      mask StyleString: popup(Rows|Columns),edit,popup(Clip Index|Clip and Warn|Generate Error)
      mask Display: disp(['Select\n' &1]);
  out : Outport
  wires:
  "Train/Data, SS2"/1 -> Legacy Cyclic Shift/1
  "Train/Data, SS2"/2 -> HT-STF Cyclic Shift/1
  Legacy Cyclic Shift/1 -> Merge Legacy/HT/1
  HT-STF Cyclic Shift/1 -> Merge Legacy/HT/2
  Merge Legacy/HT/1 -> out/1
  in/1 -> "Train/Data, SS2"/1
  "Train/Data, SS2"/3 -> HT Cyclic Shift/1
  HT Cyclic Shift/1 -> Merge Legacy/HT/3

== system ieee80211n/cyclic prefix2/Cyclic shift, SS3 ==
  in : Inport  Port=1  LatchInput=off
  HT Cyclic Shift : Selector  InputType=Matrix  Elements=[49:64 1:64]  Rows=params.cs2_HT20_ss3  Columns=-1  InputPortWidth=64
  HT-STF Cyclic Shift : Selector  InputType=Matrix  Elements=[49:64 1:64]  Rows=params.cs2_HT20_STF_ss3  Columns=-1  InputPortWidth=64
  Legacy Cyclic Shift : Selector  InputType=Matrix  Elements=[49:64 1:64]  Rows=params.cs2_Legacy_ss3  Columns=-1  InputPortWidth=64
  Merge Legacy/HT : simulink/Math Operations/Matrix Concatenation  numInports=3  catMethod=Horizontal
  "Train/Data, SS3" : S-Function  AncestorBlock=dspindex/Multiport Selector  FunctionName=sdspmultiportsel  Parameters=rowsOrCols, numOutports, flatIdxVect, flatLenVect, idxErrMode  mask(Multiport Selector){rowsOrCols=Columns, idxCellArray={params.cs2_Indices1,params.cs2_Indices2,params.cs2_Indices3}, idxErrMode=Clip Index}
      mask prompts: rowsOrCols "Select:"; idxCellArray "Indices to output:"; idxErrMode "Invalid index:"
      mask help: Output specified rows or columns to one or more output ports. The number of output ports is determined by the number of index vectors, each specified as a separate vector entry in a cell array. Indices are 1-based and need not be unique.
      mask init:
      | [numOutports, flatLenVect, flatIdxVect] = dspblkmultiportsel(idxCellArray);
      mask Help: web(dspbhelp);
      mask StyleString: popup(Rows|Columns),edit,popup(Clip Index|Clip and Warn|Generate Error)
      mask Display: disp(['Select\n' &1]);
  out : Outport
  wires:
  "Train/Data, SS3"/1 -> Legacy Cyclic Shift/1
  "Train/Data, SS3"/2 -> HT-STF Cyclic Shift/1
  Legacy Cyclic Shift/1 -> Merge Legacy/HT/1
  HT-STF Cyclic Shift/1 -> Merge Legacy/HT/2
  Merge Legacy/HT/1 -> out/1
  in/1 -> "Train/Data, SS3"/1
  "Train/Data, SS3"/3 -> HT Cyclic Shift/1
  HT Cyclic Shift/1 -> Merge Legacy/HT/3

== system ieee80211n/cyclic prefix3/Cyclic shift, SS4 ==
  in : Inport  Port=1  LatchInput=off
  HT Cyclic Shift : Selector  InputType=Matrix  Elements=[49:64 1:64]  Rows=params.cs2_HT20_ss4  Columns=-1  InputPortWidth=64
  HT-STF Cyclic Shift : Selector  InputType=Matrix  Elements=[49:64 1:64]  Rows=params.cs2_HT20_STF_ss4  Columns=-1  InputPortWidth=64
  Legacy Cyclic Shift : Selector  InputType=Matrix  Elements=[49:64 1:64]  Rows=params.cs2_Legacy_ss4  Columns=-1  InputPortWidth=64
  Merge Legacy/HT : simulink/Math Operations/Matrix Concatenation  numInports=3  catMethod=Horizontal
  "Train/Data, SS4" : S-Function  AncestorBlock=dspindex/Multiport Selector  FunctionName=sdspmultiportsel  Parameters=rowsOrCols, numOutports, flatIdxVect, flatLenVect, idxErrMode  mask(Multiport Selector){rowsOrCols=Columns, idxCellArray={params.cs2_Indices1,params.cs2_Indices2,params.cs2_Indices3}, idxErrMode=Clip Index}
      mask prompts: rowsOrCols "Select:"; idxCellArray "Indices to output:"; idxErrMode "Invalid index:"
      mask help: Output specified rows or columns to one or more output ports. The number of output ports is determined by the number of index vectors, each specified as a separate vector entry in a cell array. Indices are 1-based and need not be unique.
      mask init:
      | [numOutports, flatLenVect, flatIdxVect] = dspblkmultiportsel(idxCellArray);
      mask Help: web(dspbhelp);
      mask StyleString: popup(Rows|Columns),edit,popup(Clip Index|Clip and Warn|Generate Error)
      mask Display: disp(['Select\n' &1]);
  out : Outport
  wires:
  "Train/Data, SS4"/1 -> Legacy Cyclic Shift/1
  "Train/Data, SS4"/2 -> HT-STF Cyclic Shift/1
  Legacy Cyclic Shift/1 -> Merge Legacy/HT/1
  HT-STF Cyclic Shift/1 -> Merge Legacy/HT/2
  Merge Legacy/HT/1 -> out/1
  in/1 -> "Train/Data, SS4"/1
  "Train/Data, SS4"/3 -> HT Cyclic Shift/1
  HT Cyclic Shift/1 -> Merge Legacy/HT/3

== system ieee80211n/training sequence4/Modulator ==
  pilot : Inport  Port=1  LatchInput=off
  Frame Status Conversion1 : dspsigattribs/Frame Status Conversion  growRefPort=off  outframe=Frame-based
  "Group data for OFDM symbols " : simulink/Math Operations/Reshape  OutputDimensionality=Customize  OutputDimensions=[48 params.OFDM_LSIG_SymPerFrame]
  Group into OFDM symbols : Subsystem
      mask Display: disp('Add Pilots,\nZeros')
  Modulator 1 : Subsystem  AncestorBlock=IEEE80211a_lib/Modulator  mask(QAM Modulator-Coder.){numSymbols=48*params.OFDM_LSIG_SymPerFrame, modulation=BPSK, code=1/2, trellisStructure=poly2trellis(7, [171 133]), punctureVector=[1]}
      mask prompts: numSymbols "Number of symbols per frame:"; trellisStructure "Trellis:"; punctureVector "Puncture vector:"
      mask help: Modulator gates incoming bits so that a bank of different modulators can share the same input frame size.
      mask init:
      | % number of bits per symbol
      | switch modulation
      | 	case 'BPSK', Nb1 = 1;
      | 	case 'QPSK', Nb1 = 2;
      | 	case '16-QAM', Nb1 = 4;
      | 	case '64-QAM', Nb1 = 6;
      | end
      | 
      | modOrder = 2.^Nb1;
      | Nb = numSymbols * Nb1; % tx bits per block
      | codeRate = str2num(strvcat(code)).';
      | bitsPerBlock = Nb .* codeRate;
      | 
      | % interleaver
      | interleaverRows = 16;
      | if rem(Nb, interleaverRows)
      | 	error('Number of transmitted bits per block must be multiple of 16.')
      | end
      | interleaverCols = Nb / interleaverRows;
      | %interleaverElements = [...
      | %            2*floor( [0:Nb-1]/2 ) + ...
      | %            mod( ([0:Nb-1] + Nb - floor( interleaverRows*[0:Nb-1]/Nb ) ), 2 ) ...
      | %            + 1]';
      | interleaverElements = [...
      |             floor( [0:Nb-1] ) + ...
      |             mod( ([0:Nb-1] + Nb - floor( interleaverRows*[0:Nb-1]/Nb ) ), 1 ) ...
      |             + 1]';
      mask Display: disp(['Modulator\n' modulation ' ' code])
  Training sequence : Constant  Value=params.OFDM_LSIG_data
  out : Outport
  wires:
  Modulator 1/1(txsig) -> "Group data for OFDM symbols "/1
  Training sequence/1 -> Frame Status Conversion1/1
  Frame Status Conversion1/1 -> Modulator 1/1(txdata)
  "Group data for OFDM symbols "/1 -> Group into OFDM symbols/2(in)
  Group into OFDM symbols/1(out) -> out/1
  pilot/1 -> Group into OFDM symbols/1(in1)

== system ieee80211n/training sequence4/Modulator1 ==
  pilot : Inport  Port=1  LatchInput=off
  Frame Status Conversion1 : dspsigattribs/Frame Status Conversion  growRefPort=off  outframe=Frame-based
  "Group data for OFDM symbols " : simulink/Math Operations/Reshape  OutputDimensionality=Customize  OutputDimensions=[48 params.OFDM_HTSIG_SymPerFrame]
  Group into OFDM symbols : Subsystem
      mask Display: disp('Add Inv.\nPilots')
  Modulator 2 : Subsystem  AncestorBlock=IEEE80211a_lib/Modulator  mask(QAM Modulator-Coder.){numSymbols=48*params.OFDM_HTSIG_SymPerFrame, modulation=BPSK, code=1/2, trellisStructure=poly2trellis(7, [171 133]), punctureVector=[1]}
      mask prompts: numSymbols "Number of symbols per frame:"; trellisStructure "Trellis:"; punctureVector "Puncture vector:"
      mask help: Modulator gates incoming bits so that a bank of different modulators can share the same input frame size.
      mask init: same as ieee80211n/training sequence4/Modulator/Modulator 1
      mask Display: disp(['Modulator\n' modulation ' ' code])
  Training sequence : Constant  Value=params.OFDM_HTSIG_data
  out : Outport
  wires:
  Modulator 2/1(txsig) -> "Group data for OFDM symbols "/1
  Training sequence/1 -> Frame Status Conversion1/1
  Frame Status Conversion1/1 -> Modulator 2/1(txdata)
  "Group data for OFDM symbols "/1 -> Group into OFDM symbols/2(in)
  Group into OFDM symbols/1(out) -> out/1
  pilot/1 -> Group into OFDM symbols/1(in1)

== system ieee80211n/training sequence4/Pilots ==
  PN Sequence Generator : commseqgen2/PN Sequence Generator  poly=[1 0 0 0 1 0 0 1]  ini_sta=[1 1 1 1 1 1 1]  shift=0  Ts=params.blockPeriod/(params.OFDM_LSIG_SymPerFrame+params.OFDM_HTSIG_SymPerFrame+params.OFDMSymPerFrame)  frameBased=on  sampPerFrame=(params.OFDM_LSIG_SymPerFrame+params.OFDM_HTSIG_SymPerFrame+params.OFDMSymPerFrame)  reset=off
  Reshape : S-Function  AncestorBlock=simulink/Math Operations/Reshape  FunctionName=sreshape  Parameters=OutputDimensionality, OutputDimensions  mask(Reshape){OutputDimensionality=Row vector, OutputDimensions=[1,1]}
      mask prompts: OutputDimensionality "Output dimensionality:"; OutputDimensions "Output dimensions:"
      mask help:
      | Change the dimensions of a vector or matrix input signal. Output
      |  - a one-dimensional array (vector),
      |  - a column vector (Mx1 matrix),
      |  - a row vector (1xN matrix), or
      |  - a matrix or vector with specified dimensions, e.g., [M, N] or [W].
      mask init:
      | s = reshapemask(gcb,'init');
      mask StyleString: popup(1-D array|Column vector|Row vector|Customize),edit
      mask CallbackString: reshapemask(gcb,'cbDimensionality')|
      mask Display: plot(s.x1,s.y1,s.xc,s.yc);
  Unipolar to Bipolar Converter : Subsystem  AncestorBlock=|  mask(Unipolar to Bipolar Converter){M=2, polarity=Negative}
      | commutil2/Unipolar to
      | Bipolar
      | Converter
      mask prompts: M "M-ary number:"
      mask help: Convert a unipolar signal in the range [0, M-1], where M is the M-ary number, into a bipolar signal.
      mask init:
      | if strcmp(polarity, 'Negative')
      |    pole = -1;
      | else
      |    pole = 1;
      | end
      mask Help: helpview(commbhelp);
      mask StyleString: edit,popup(Positive|Negative)
      mask Display: disp('Unipolar to\nBipolar\nConverter');
  out : Outport
  wires:
  Reshape/1 -> out/1
  Unipolar to Bipolar Converter/1(Out1) -> Reshape/1
  PN Sequence Generator/1 -> Unipolar to Bipolar Converter/1(In1)

== system ieee80211n/training sequence4/training sequence ==
  Frame Status Conversion1 : dspsigattribs/Frame Status Conversion  growRefPort=off  outframe=Frame-based
  Training sequence : Constant  Value=repmat(params.long_training_seq, [1 params.OFDM_LLTF_SymPerFrame])
  out : Outport
  wires:
  Training sequence/1 -> Frame Status Conversion1/1
  Frame Status Conversion1/1 -> out/1
